simulink model "PowerFlow_SUSAN_Vector"  (R2022b)
settings: Solver=FixedStepAuto  StartTime=0.0  StopTime=10  FixedStep=0.02  RelTol=1e-3
libraries: Lib_EMTAT x17
settings Model: Creator=sbianco1  LastModifiedBy=sbianco1
settings SolverCC: AlgebraicLoopSolver=TrustRegion
settings DebuggingCC: UnconnectedInputMsg=warning  UnconnectedOutputMsg=warning  UnconnectedLineMsg=warning  SFMachineParentedDataDiag=warning
settings ModelReferenceCC: EnableRefExpFcnMdlSchedulingChecks=on
settings RTWCC: DLArmComputeVersion=19.05

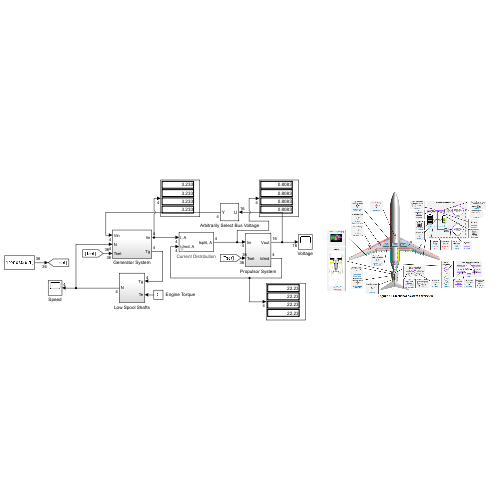
[thumbnail: Simulink's stored preview of the top-level diagram]
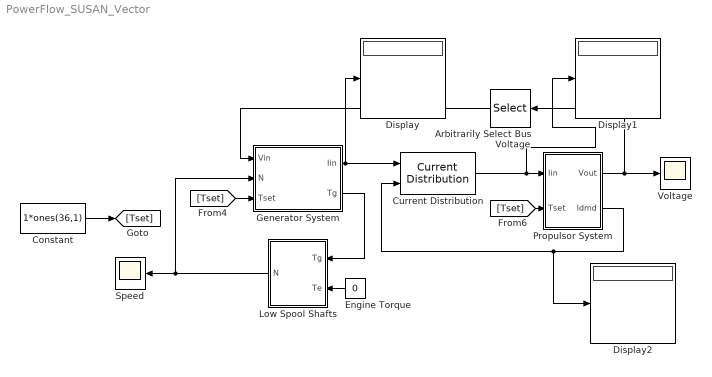
== system PowerFlow_SUSAN_Vector ==
  Arbitrarily Select Bus Voltage : Selector  InputPortWidth=16  IndexOptions=Index vector (dialog)  Indices=[1 5 9 13]  OutputSizes=1
  Constant : Constant  Value=1*ones(36,1)
  Current Distribution : Lib_EMTAT/Components/Power Flow/Current Distribution
      settings: AttributesFormatString=Current Distribution  SourceProductName=EMTAT
  Display : Display
  Display1 : Display
  Display2 : Display
  Engine Torque : Constant  Value=0
  Generator System : Subsystem
  Low Spool Shafts : Subsystem
  Propulsor System : Subsystem
  Speed : Scope
  Voltage : Scope
  wires:
  Engine Torque/1 -> Low Spool Shafts/2(Te)
  Generator System/2(Tg) -> Low Spool Shafts/1(Tg)
  Propulsor System/1(Vout) -> Voltage/1, Arbitrarily Select Bus Voltage/1
  Constant/1 -> [Tset]
  [Tset] -> Generator System/3(Tset)
  Low Spool Shafts/1(N) -> Speed/1, Generator System/2(N)
  Generator System/1(Iin) -> Current Distribution/1, Display/1
  Current Distribution/1 -> Display1/1, Propulsor System/1(Iin)
  [Tset] -> Propulsor System/2(Tset)
  Propulsor System/2(Idmd) -> Display2/1, Current Distribution/2
  Arbitrarily Select Bus Voltage/1 -> Generator System/1(Vin)

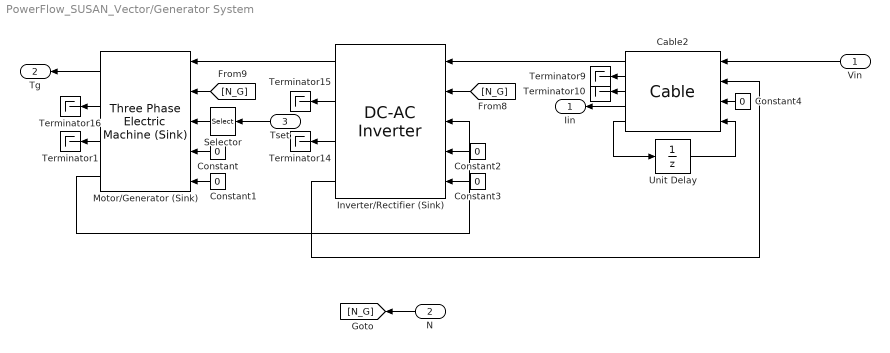
== system PowerFlow_SUSAN_Vector/Generator System ==
  Vin : Inport
  N : Inport  Port=2
  Tset : Inport  Port=3
  Cable2 : Lib_EMTAT/Components/Power Flow/Cable  R=0.2
      settings: SourceProductName=EMTAT
  Constant{,1..4} (5 alike) : Constant  Value=0
  Inverter/Rectifier (Sink) : Lib_EMTAT/Components/Power Flow/DC-AC Inverter  X_C_VoltageInVec_M=[0 1000]  Y_C_RMSCurrentOutVec_M=[0 1000]  T_C_PowLossArray_M=zeros(2)  K_e=0.0503  FM=0  Plosslim=0
      settings: SourceProductName=EMTAT
  Motor/Generator (Sink) : Lib_EMTAT/Components/Power Flow/Three Phase Electric Machine (Sink)  X_C_SpeedVec_M=[0 100 1000 5000]  Y_C_TorqueVec_M=[0 10 100 150]  T_C_EffArray_M=0.99*ones(4,4)  FM=0
      settings: SourceProductName=EMTAT
  Selector : Selector  InputPortWidth=36  IndexOptions=Index vector (dialog)  Indices=[33:36]  OutputSizes=1
  Terminator{1,9..10,14..16} (6 alike) : Terminator
  Unit Delay : UnitDelay  SampleTime=-1  HasFrameUpgradeWarning=on
  Iin : Outport
  Tg : Outport  Port=2
  wires:
  Unit Delay/1 -> Cable2/4
  Inverter/Rectifier (Sink)/2 -> Terminator15/1
  Motor/Generator (Sink)/4 -> Inverter/Rectifier (Sink)/3
  Inverter/Rectifier (Sink)/4 -> Cable2/2
  Cable2/1 -> Inverter/Rectifier (Sink)/1
  Motor/Generator (Sink)/1 -> Tg/1
  Cable2/5 -> Unit Delay/1
  [N_G] -> Inverter/Rectifier (Sink)/2
  Motor/Generator (Sink)/2 -> Terminator16/1
  Inverter/Rectifier (Sink)/3 -> Terminator14/1
  Cable2/3 -> Terminator10/1
  Inverter/Rectifier (Sink)/1 -> Motor/Generator (Sink)/1
  [N_G] -> Motor/Generator (Sink)/2
  Cable2/2 -> Terminator9/1
  Vin/1 -> Cable2/1
  Cable2/4 -> Iin/1
  N/1 -> [N_G]
  Selector/1 -> Motor/Generator (Sink)/3
  Motor/Generator (Sink)/3 -> Terminator1/1
  Tset/1 -> Selector/1
  Constant/1 -> Motor/Generator (Sink)/4
  Constant1/1 -> Motor/Generator (Sink)/5
  Constant2/1 -> Inverter/Rectifier (Sink)/4
  Constant3/1 -> Inverter/Rectifier (Sink)/5
  Constant4/1 -> Cable2/3

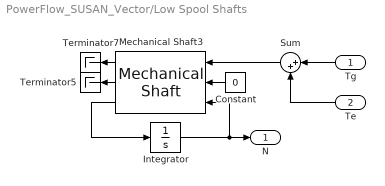
== system PowerFlow_SUSAN_Vector/Low Spool Shafts ==
  Tg : Inport
  Te : Inport  Port=2
  Constant : Constant  Value=0
  Integrator : Integrator  InitialCondition=5000
  Mechanical Shaft3 : Lib_EMTAT/Components/Power Flow/Mechanical Shaft  J=0.01  B=0.001
      settings: SourceProductName=EMTAT
  Sum : Sum  Inputs=|++
  Terminator5 : Terminator
  Terminator7 : Terminator
  N : Outport
  wires:
  Mechanical Shaft3/2 -> Terminator5/1
  Integrator/1 -> Mechanical Shaft3/3, N/1
  Tg/1 -> Sum/1
  Te/1 -> Sum/2
  Sum/1 -> Mechanical Shaft3/1
  Mechanical Shaft3/1 -> Terminator7/1
  Mechanical Shaft3/3 -> Integrator/1
  Constant/1 -> Mechanical Shaft3/2

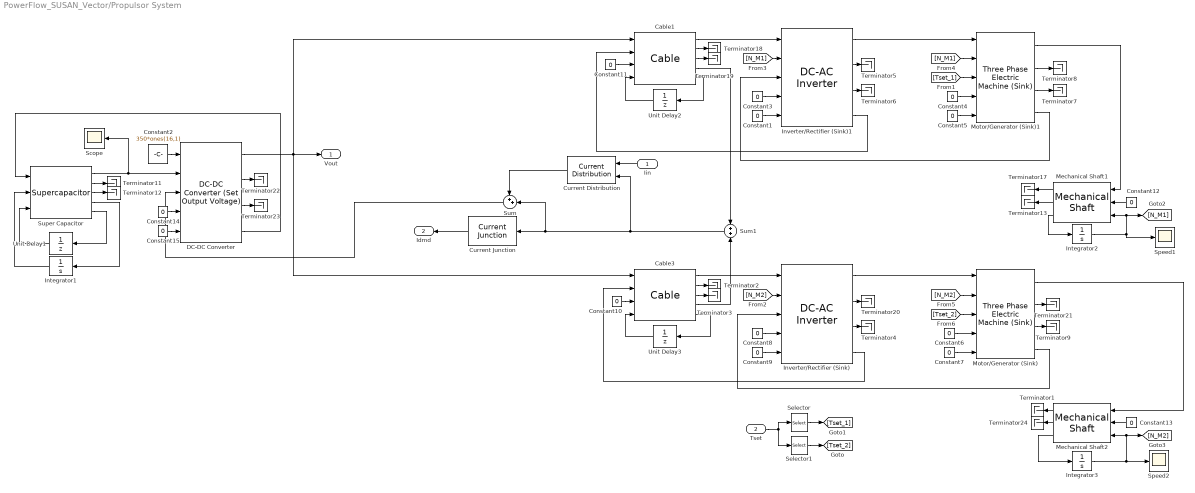
== system PowerFlow_SUSAN_Vector/Propulsor System ==
  Iin : Inport
  Tset : Inport  Port=2
  Cable1 : Lib_EMTAT/Components/Power Flow/Cable  R=0.2
      settings: SourceProductName=EMTAT
  Cable3 : Lib_EMTAT/Components/Power Flow/Cable  R=0.2
      settings: SourceProductName=EMTAT
  Constant{1,3..15} (14 alike) : Constant  Value=0
  Constant2 : Constant  Value=350*ones(16,1)
  Current Distribution : Lib_EMTAT/Components/Power Flow/Current Distribution
      settings: AttributesFormatString=Current Distribution  SourceProductName=EMTAT
  Current Junction : Lib_EMTAT/Components/Power Flow/Current Junction  Nb=4
      settings: AttributesFormatString=Current Junction  SourceProductName=EMTAT
  DC-DC Converter : Lib_EMTAT/Components/Power Flow/DC-DC Converter (Set Output Voltage)  X_Vin_VoltageVec_M=[0 100 1000 5000]  Y_Iout_CurrentVec_M=[0 10 100 150]  T_C_PlossArray_M=0.98*ones(4,4)  FM=0  Plosslim=0
      settings: SourceProductName=EMTAT
  Integrator1 : Integrator  InitialCondition=150
  Integrator2 : Integrator  InitialCondition=2000
  Integrator3 : Integrator  InitialCondition=2000
  Inverter/Rectifier (Sink) : Lib_EMTAT/Components/Power Flow/DC-AC Inverter  X_C_VoltageInVec_M=[0 1000]  Y_C_RMSCurrentOutVec_M=[0 1000]  T_C_PowLossArray_M=zeros(2)  K_e=0.0503  FM=0  Plosslim=0
      settings: SourceProductName=EMTAT
  Inverter/Rectifier (Sink)1 : Lib_EMTAT/Components/Power Flow/DC-AC Inverter  X_C_VoltageInVec_M=[0 1000]  Y_C_RMSCurrentOutVec_M=[0 1000]  T_C_PowLossArray_M=zeros(2)  K_e=0.0503  FM=0  Plosslim=0
      settings: SourceProductName=EMTAT
  Mechanical Shaft1 : Lib_EMTAT/Components/Power Flow/Mechanical Shaft  J=0.01  B=0.001
      settings: SourceProductName=EMTAT
  Mechanical Shaft2 : Lib_EMTAT/Components/Power Flow/Mechanical Shaft  J=0.01  B=0.001
      settings: SourceProductName=EMTAT
  Motor/Generator (Sink) : Lib_EMTAT/Components/Power Flow/Three Phase Electric Machine (Sink)  X_C_SpeedVec_M=[0 100 1000 5000]  Y_C_TorqueVec_M=[0 10 100 150]  T_C_EffArray_M=0.99*ones(4,4)  FM=0
      settings: SourceProductName=EMTAT
  Motor/Generator (Sink)1 : Lib_EMTAT/Components/Power Flow/Three Phase Electric Machine (Sink)  X_C_SpeedVec_M=[0 100 1000 5000]  Y_C_TorqueVec_M=[0 10 100 150]  T_C_EffArray_M=0.99*ones(4,4)  FM=0
      settings: SourceProductName=EMTAT
  Scope : Scope
  Selector : Selector  InputPortWidth=36  IndexOptions=Index vector (dialog)  Indices=[1:16]  OutputSizes=1
  Selector1 : Selector  InputPortWidth=36  IndexOptions=Index vector (dialog)  Indices=[17:32]  OutputSizes=1
  Speed1 : Scope
  Speed2 : Scope
  Sum : Sum  Inputs=++|
  Sum1 : Sum
  Super Capacitor : Lib_EMTAT/Components/Power Flow/Supercapacitor  C=130  ESR=0.02  TSE=200  BlkNm=double(gcb)
      settings: SourceProductName=EMTAT
  Terminator{1..9,11..13,17..24} (20 alike) : Terminator
  Unit Delay1 : UnitDelay  SampleTime=-1  HasFrameUpgradeWarning=on
  Unit Delay2 : UnitDelay  SampleTime=-1  HasFrameUpgradeWarning=on
  Unit Delay3 : UnitDelay  SampleTime=-1  HasFrameUpgradeWarning=on
  Vout : Outport
  Idmd : Outport  Port=2
  wires:
  Mechanical Shaft2/3 -> Integrator3/1
  [Tset_1] -> Motor/Generator (Sink)1/3
  [N_M2] -> Motor/Generator (Sink)/2
  DC-DC Converter/1 -> Cable1/1, Vout/1, Cable3/1
  Mechanical Shaft1/3 -> Integrator2/1
  Motor/Generator (Sink)1/4 -> Inverter/Rectifier (Sink)1/3
  Super Capacitor/4 -> Integrator1/1
  Super Capacitor/1 -> Scope/1, DC-DC Converter/2
  Cable3/1 -> Inverter/Rectifier (Sink)/1
  [N_M1] -> Motor/Generator (Sink)1/2
  Unit Delay2/1 -> Cable1/4
  Cable3/2 -> Terminator2/1
  DC-DC Converter/4 -> Super Capacitor/1
  Sum1/1 -> Current Junction/1, Sum/2, Current Distribution/2
  Integrator2/1 -> [N_M1], Mechanical Shaft1/3, Speed1/1
  Cable1/1 -> Inverter/Rectifier (Sink)1/1
  [N_M1] -> Inverter/Rectifier (Sink)1/2
  Cable3/5 -> Unit Delay3/1
  Inverter/Rectifier (Sink)1/1 -> Motor/Generator (Sink)1/1
  Inverter/Rectifier (Sink)/3 -> Terminator4/1
  Super Capacitor/2 -> Terminator11/1
  Cable3/4 -> Sum1/2
  Integrator3/1 -> Speed2/1, [N_M2], Mechanical Shaft2/3
  Inverter/Rectifier (Sink)/1 -> Motor/Generator (Sink)/1
  Inverter/Rectifier (Sink)/2 -> Terminator20/1
  Cable1/3 -> Terminator19/1
  Motor/Generator (Sink)/4 -> Inverter/Rectifier (Sink)/3
  Unit Delay3/1 -> Cable3/4
  Inverter/Rectifier (Sink)1/4 -> Cable1/2
  Integrator1/1 -> Super Capacitor/2
  Cable1/5 -> Unit Delay2/1
  Inverter/Rectifier (Sink)1/3 -> Terminator6/1
  Super Capacitor/5 -> Unit Delay1/1
  Unit Delay1/1 -> Super Capacitor/3
  Cable1/4 -> Sum1/1
  Constant2/1 -> DC-DC Converter/1
  Motor/Generator (Sink)1/2 -> Terminator8/1
  Cable3/3 -> Terminator3/1
  Motor/Generator (Sink)/1 -> Mechanical Shaft2/1
  Cable1/2 -> Terminator18/1
  Super Capacitor/3 -> Terminator12/1
  Motor/Generator (Sink)/2 -> Terminator21/1
  Inverter/Rectifier (Sink)/4 -> Cable3/2
  [N_M2] -> Inverter/Rectifier (Sink)/2
  DC-DC Converter/2 -> Terminator22/1
  DC-DC Converter/3 -> Terminator23/1
  [Tset_2] -> Motor/Generator (Sink)/3
  Inverter/Rectifier (Sink)1/2 -> Terminator5/1
  Motor/Generator (Sink)1/1 -> Mechanical Shaft1/1
  Selector/1 -> [Tset_1]
  Selector1/1 -> [Tset_2]
  Tset/1 -> Selector/1, Selector1/1
  Mechanical Shaft2/1 -> Terminator1/1
  Mechanical Shaft2/2 -> Terminator24/1
  Mechanical Shaft1/2 -> Terminator13/1
  Mechanical Shaft1/1 -> Terminator17/1
  Motor/Generator (Sink)1/3 -> Terminator7/1
  Motor/Generator (Sink)/3 -> Terminator9/1
  Current Junction/1 -> Idmd/1
  Iin/1 -> Current Distribution/1
  Current Distribution/1 -> Sum/1
  Sum/1 -> DC-DC Converter/3
  Constant3/1 -> Inverter/Rectifier (Sink)1/4
  Constant1/1 -> Inverter/Rectifier (Sink)1/5
  Constant4/1 -> Motor/Generator (Sink)1/4
  Constant5/1 -> Motor/Generator (Sink)1/5
  Constant6/1 -> Motor/Generator (Sink)/4
  Constant7/1 -> Motor/Generator (Sink)/5
  Constant8/1 -> Inverter/Rectifier (Sink)/4
  Constant9/1 -> Inverter/Rectifier (Sink)/5
  Constant10/1 -> Cable3/3
  Constant11/1 -> Cable1/3
  Constant12/1 -> Mechanical Shaft1/2
  Constant13/1 -> Mechanical Shaft2/2
  Constant14/1 -> DC-DC Converter/4
  Constant15/1 -> DC-DC Converter/5
